simulink model "xEMU_SimulationModel3_rule1"  (R2017b)
settings: Solver=ode4  StartTime=0.0  StopTime=8192  FixedStep=0.01  RelTol=1e-3
undefined symbols (not defined in the file): a1, a2, a3, a4, ACO, BAT, Battery, DCT, DRT, EMS, ENV, Fahrzyklus_VS_modell, height_BAT, leistung, lib_bat, Maximum, Maximum_position, Num_cells, P_FC_max_long, P_FC_min_long, P_FC_step_max, Pbat_charge_max, Pbat_discharge_max, Pfc_max, Pfc_min, SOC_tar, time_peaks, TRM, velocity_peaks
libraries: simulink x5
(part 9 of 15)

== system xEMU_SimulationModel3_rule1/Battery (BAT)_komplex/Subsystem/ElectricalCircuit/Cellelement_Elem1/Rmphn_Elem2 ==
  T : Inport
  SoC : Inport  Port=2
  Object : Lookup_n-D  BreakpointsForDimension1=[10 25 35 45]  BreakpointsForDimension2=[0 5 10 15 20 25 30 35 40 45 50 55 60 65 70 75 80 85 90 95 100]  Table=[0.000268122505057072 0.00046251136129643 0.000643717837942068 0.000610386454678535 0.00045685192101357 0.000388035738603161 0.000336878735294759 0.000333375986684024 0.000321108800701806 0.000318973974892479 0.000303391249635262 0.000303204281029518 0.000297787044358361 0.000300249237624058 0.000298711247305386 0.000297350259051319 0.000301859274253576 0.000313998160496946 0.000341701603840128 0.000417691070242408 0.000417689978158318;0.105441120159789 0.00096755218954419 0.000529404764033394 0.000354619127347272 0.000284612269108788 0.000251721272272473 0.000252493664676402 0.000230094357795404 0.000207521825021393 0.000190441374899878 0.000178637719620051 0.000177529745884289 0.000175505765036172 0.000173031403485662 0.000172679629835472 0.000166312191557979 0.00017401143861351 0.000199341075567154 0.000255464654695431 0.00070692540667571 0.00353955118648807;0.00118157328513432 0.000748992447788816 0.000451818583841663 0.000290076474209044 0.000194362347991163 0.000143830566471477 9.92210097897263e-05 7.40619477978304e-05 4.40775921405744e-05 4.31116426933342e-05 4.09849161117321e-05 4.10541548999212e-05 3.8267267500746e-05 3.63092794956421e-05 4.14869060972538e-05 4.49104540893705e-05 4.59660513161652e-05 4.86952421140127e-05 4.94130500198532e-05 0.000127040319833249 0.000525588842740708;0.000669172169658894 0.000379477976380309 0.000231415435891332 0.000136838362951624 9.37210144790436e-05 0.00022453139764744 0.000261681601370784 0.000275717918924215 0.000343387485925263 0.000309569655761013 0.000327723280548032 0.000346361466696158 0.000355248627933966 0.000383511648660796 0.000762747032591511 0.000482937839790971 0.000437851512368699 0.000453348455645594 0.000469989279725756 0.000620721089927547 0.000273243452522911]  ExtrapMethod=Clip  RndMeth=Simplest  InputSameDT=on
  Tau : Lookup_n-D  BreakpointsForDimension1=[10 25 35 45]  BreakpointsForDimension2=[0 5 10 15 20 25 30 35 40 45 50 55 60 65 70 75 80 85 90 95 100]  Table=[0.000141955461410132 0.000108259964906405 7.80774844155858e-05 0.000101831536112891 0.000107975924751293 0.000108564940513868 0.000111641696811859 0.000113299614321864 0.000112465051722286 9.97340191359942e-05 0.000108640252661311 0.000108951310987874 0.000109254278947402 0.000109366925113906 0.000111301823135108 0.000118543460124368 0.000128410735701329 0.00012644454704452 0.000133838402973526 0.000136136544113434 9.82118308687161e-05;1.44148342133733e-06 1.04132356690357e-05 1.53197904992227e-05 1.58298746298682e-05 1.04100480339941e-05 4.49161696524291e-06 7.51385938203224e-07 1.19998828380278e-06 1.7484531583263e-06 2.24727945021076e-06 2.85288799447317e-06 2.3982374887958e-06 2.5543004122239e-06 2.84146194349035e-06 3.29845050624667e-06 4.36998458930454e-06 5.14859008826645e-06 5.1127506304825e-06 3.70215417911144e-06 1.08280333595243e-06 -3.40186367207846e-08;1e-07 1e-07 2.31775917823548e-07 5.9109862793901e-07 1.41930407022604e-06 2.53894683649514e-06 4.87494541206615e-06 8.66810441183524e-06 1.68823285933497e-05 1.74360926052191e-05 1.75424559454703e-05 1.6623303179158e-05 1.86276926994013e-05 1.90117503381529e-05 1.99503323044723e-05 2.10803940917103e-05 2.22552249334782e-05 2.42579904812111e-05 2.41449451303551e-05 1.01960705344891e-05 8.23637353204037e-07;1e-07 1e-07 1.00006555422865e-07 1.76638744052027e-07 1.40361049557971e-06 1.80241729343279e-06 1.14320296152634e-06 6.20353351220257e-07 3.57247497379756e-07 2.03111810542261e-07 1.41684357923681e-07 1.00689263423425e-07 1.01438254958135e-07 1.04869717402227e-07 1e-07 1e-07 1.00012811085513e-07 1.05628050575502e-07 2.21581233292744e-07 7.96773138822328e-07 2.25608914428729e-06]  ExtrapMethod=Clip  RndMeth=Simplest  InputSameDT=on
  tag scope: ID4_ObjCT=global, ID4_ObjMP=global
  wires:
  Object/1 -> [ID4_ObjCT]
  T/1 -> Object/1, Tau/1
  SoC/1 -> Object/2, Tau/2
  Tau/1 -> [ID4_ObjMP]

== system xEMU_SimulationModel3_rule1/Battery (BAT)_komplex/Subsystem/ElectricalCircuit/Cellelement_Elem1/Rmphn_Elem3 ==
  T : Inport
  SoC : Inport  Port=2
  Object : Lookup_n-D  BreakpointsForDimension1=[10 25 35 45]  BreakpointsForDimension2=[0 5 10 15 20 25 30 35 40 45 50 55 60 65 70 75 80 85 90 95 100]  Table=[0.000268122505057072 0.00046251136129643 0.000643717837942068 0.000610386454678535 0.00045685192101357 0.000388035738603161 0.000336878735294759 0.000333375986684024 0.000321108800701806 0.000318973974892479 0.000303391249635262 0.000303204281029518 0.000297787044358361 0.000300249237624058 0.000298711247305386 0.000297350259051319 0.000301859274253576 0.000313998160496946 0.000341701603840128 0.000417691070242408 0.000417689978158318;0.105441120159789 0.00096755218954419 0.000529404764033394 0.000354619127347272 0.000284612269108788 0.000251721272272473 0.000252493664676402 0.000230094357795404 0.000207521825021393 0.000190441374899878 0.000178637719620051 0.000177529745884289 0.000175505765036172 0.000173031403485662 0.000172679629835472 0.000166312191557979 0.00017401143861351 0.000199341075567154 0.000255464654695431 0.00070692540667571 0.00353955118648807;0.00118157328513432 0.000748992447788816 0.000451818583841663 0.000290076474209044 0.000194362347991163 0.000143830566471477 9.92210097897263e-05 7.40619477978304e-05 4.40775921405744e-05 4.31116426933342e-05 4.09849161117321e-05 4.10541548999212e-05 3.8267267500746e-05 3.63092794956421e-05 4.14869060972538e-05 4.49104540893705e-05 4.59660513161652e-05 4.86952421140127e-05 4.94130500198532e-05 0.000127040319833249 0.000525588842740708;0.000669172169658894 0.000379477976380309 0.000231415435891332 0.000136838362951624 9.37210144790436e-05 0.00022453139764744 0.000261681601370784 0.000275717918924215 0.000343387485925263 0.000309569655761013 0.000327723280548032 0.000346361466696158 0.000355248627933966 0.000383511648660796 0.000762747032591511 0.000482937839790971 0.000437851512368699 0.000453348455645594 0.000469989279725756 0.000620721089927547 0.000273243452522911]  ExtrapMethod=Clip  RndMeth=Simplest  InputSameDT=on
  Tau : Lookup_n-D  BreakpointsForDimension1=[10 25 35 45]  BreakpointsForDimension2=[0 5 10 15 20 25 30 35 40 45 50 55 60 65 70 75 80 85 90 95 100]  Table=[0.000529292712630017 0.000351382846491099 0.000177810480944207 7.79403990960714e-05 6.81569541336992e-05 5.91040264946733e-05 5.28632407026636e-05 3.86685791728393e-05 3.41763608587333e-05 3.90598295370642e-05 3.33343419869487e-05 3.31788561799858e-05 3.72164662468986e-05 3.7819623059679e-05 3.92982398452099e-05 3.90459805088247e-05 3.94718130171938e-05 5.00153524126515e-05 5.77919815211187e-05 6.30552678733864e-05 0.000194648514008883;5.50411647601813e-06 3.52318210856722e-05 3.07460510072176e-05 2.88125567107061e-05 3.20934600958392e-05 3.98196491910542e-05 4.70065039136467e-05 4.16667581912915e-05 3.8766931651523e-05 3.73480760967852e-05 3.75368686771652e-05 3.79235652388832e-05 3.82366651889809e-05 3.77564206326725e-05 3.77697732369037e-05 3.92608610070005e-05 4.09722828338765e-05 4.41317395295982e-05 4.92214251960363e-05 4.91775019181766e-05 2.37762839960349e-06;2.79835750709802e-05 2.77652269593851e-05 2.59170689623705e-05 2.30145827749915e-05 2.06316035856238e-05 1.73996721774708e-05 1.69083782724042e-05 1.54723392916681e-05 1.54113892744735e-05 1.29818644067297e-05 1.18550990934711e-05 1.13907271327181e-05 1.16978907519504e-05 1.16639401630886e-05 6.99591929291379e-06 5.60005970916921e-06 6.20584876015212e-06 7.3565325766759e-06 1.5073212633788e-05 1.73520798215733e-05 1.32236073562572e-05;1.88609117562345e-05 1.56983515705563e-05 1.13522959669512e-05 8.43457227299759e-06 5.05996632935698e-06 1.95249155023466e-07 1.76960347573296e-07 1.67193948116137e-07 1.13790792161104e-07 1.54842321962181e-07 1.59787929658381e-07 1.79195596001854e-07 1.93858272726632e-07 1.959423113329e-07 1.0263240562418e-07 1.4811966509328e-07 2.15247631988995e-07 2.26942289219901e-07 2.61537981718251e-07 6.32640243600376e-07 6.94233450436108e-06]  ExtrapMethod=Clip  RndMeth=Simplest  InputSameDT=on
  tag scope: ID5_ObjCT=global, ID5_ObjMP=global
  wires:
  Object/1 -> [ID5_ObjCT]
  T/1 -> Object/1, Tau/1
  SoC/1 -> Object/2, Tau/2
  Tau/1 -> [ID5_ObjMP]

== system xEMU_SimulationModel3_rule1/Battery (BAT)_komplex/Subsystem/ElectricalCircuit/Cellelement_Elem1/SphericalDiffusion_Elem4 ==
  T : Inport
  SoC : Inport  Port=2
  Object : Lookup_n-D  BreakpointsForDimension1=[10 25 35 45]  BreakpointsForDimension2=[0 5 10 15 20 25 30 35 40 45 50 55 60 65 70 75 80 85 90 95 100]  Table=[0.00430313409541137 0.00258316736106707 0.000909014786104972 1.18545506602962e-05 4.38366113693087e-05 8.77044399626091e-05 5.79079218847818e-05 0.000150514980577749 9.33787733777284e-05 0.000170587402323895 9.16912408369071e-05 0.000169973923190152 0.0010864171289951 0.0010168205375952 5.17594049421499e-05 5.25039764358344e-05 7.13543000736091e-05 9.72674277356414e-05 0.000262863352777946 6.70953684616619e-05 6.70949924803742e-05;0.00202864818193681 0.000693578367286168 0.000184380393678643 0.000403287595693715 0.000127662300666302 4.76087328882778e-05 0.000131120918827474 0.000337353209406746 6.4631465676567e-05 0.000123474566106843 8.04635241293952e-05 0.000162451054715727 0.000533166288895852 7.92410317103854e-05 8.48020493836965e-05 5.24883118428218e-05 2.91838096707873e-05 0.000114184116093498 0.000126907742418507 1.73539545684722e-05 1.73540061952083e-05;0.00103112903028711 4.07365124309712e-05 3.42260849887195e-05 6.30654379412048e-05 0.00016624324470566 9.00400976993266e-05 6.22392485080555e-05 0.00029158679942256 5.17588808408712e-05 0.000140058855505779 9.00232650693359e-05 8.92568237263442e-05 5.25312934291685e-05 8.92665162019484e-05 5.22566775637766e-05 0.000100524062848508 0.000141278584594374 0.000119351605629175 0.000299281628089723 0.00026149287385724 0.000261489941349852;0.000621026899352884 5.60368895320236e-05 3.18742117279188e-05 4.05885789487214e-05 3.91921275086055e-05 7.19709567229367e-05 0.000189740995702097 0.000253909950020527 0.000269517412491939 0.000277425145551863 0.000296662547586413 0.000291880241147839 0.00023830686533216 0.000175595640657073 0.000217368080740519 0.000222023403173585 0.000184231812431194 0.0002351483403811 0.000169922728749226 0.000268921139693127 0.00026891992725363]  ExtrapMethod=Clip  RndMeth=Simplest  InputSameDT=on
  Tau : Lookup_n-D  BreakpointsForDimension1=[10 25 35 45]  BreakpointsForDimension2=[0 5 10 15 20 25 30 35 40 45 50 55 60 65 70 75 80 85 90 95 100]  Table=[1115.38517775812 684.657648467646 263.177144419379 3.81744728467607 15.1293962439251 30.9953004856576 20.1374386136996 46.1976468763129 24.3342331115565 36.3078360953177 16.0981709839934 33.6491773394059 348.511561205692 928.37037442187 12.4483953448915 9.53242773674869 11.3400431038893 14.0420254456782 35.6196175844955 5.18032976962323 5.18029939245667;436.05721547597 178.788072232168 55.3194371233784 131.268654128176 44.6888118749279 17.3143772686759 44.9030974055553 105.796849607155 16.2649172847531 26.9015680841646 14.7268525811286 49.9719994898928 229.019627822504 43.8344050464637 18.918379680171 9.58535878036457 4.50330552785554 16.5919956763023 17.1024869877413 1.47841513907696 1.47839793558041;224.745225665794 10.4369473657352 10.1100156485882 20.6404452475675 59.9999171658416 33.7203018879835 22.2490337021504 92.460322726672 13.7046257706988 30.9800391075748 16.5730721535485 17.2353609039221 29.7188074063282 41.244592651443 11.3392979117728 18.0373016773353 22.5168418427195 17.3027128393532 40.2554135594826 22.7934252028777 22.7929913223903;132.312832757629 14.8466722088249 9.50749347362856 13.5149063331701 14.1435250573307 27.3268542237605 70.5271372880475 83.4077698431377 73.7985753726319 61.9682148848562 55.6945245498801 65.449708470853 159.041871284961 66.2172719242345 46.1341060367769 39.5262197327382 29.1421856819277 33.9899451331094 21.9811449727135 21.6842433004828 1.05441000209685]  ExtrapMethod=Clip  RndMeth=Simplest  InputSameDT=on
  tag scope: ID6_ObjR=global, ID6_ObjTau=global
  wires:
  Object/1 -> [ID6_ObjR]
  T/1 -> Object/1, Tau/1
  SoC/1 -> Object/2, Tau/2
  Tau/1 -> [ID6_ObjTau]
